simulink model "ModeAdjust"  (R2018b)
settings: Solver=FixedStepDiscrete  StartTime=0.0  StopTime=inf  FixedStep=0.01  RelTol=1e-3
undefined symbols (not defined in the file or in its folder): IfKeSMSbSeatMovBkRclnEnable_Val, IfKeSMSbSeatMovFrwdBkwdEnable_Val, IfKeSMSbSeatMovFtrstEnable_Val, IfKeSMSbSeatMovHdrstFrwdBkwdEnable_Val, IfKeSMSbSeatMovHdUpwdDnwdEnable_Val, IfKeSMSbSeatMovLgrstEnable_Val, IfKeSMSbSeatMovLtwdRtwdEnable_Val, IfVeSMSeStNumConfig, KeSMSbArmscreenMovEnable_Val, KeSMSbSeatMovLgrstExpdEnable_Val, KeSMSuFirstRwStBackPosDelta_Val, KeSMSuFirstRwStBackPosTolr_Val, KeSMSuFirstRwStCushFrntPosDelta_Val, KeSMSuFirstRwStCushFrntPosTolr_Val, KeSMSuFirstRwStCushRePosDelta_Val, KeSMSuFirstRwStCushRePosTolr_Val, KeSMSuFirstRwStFootrestPosDelta_Val, KeSMSuFirstRwStFootrestPosTolr_Val, KeSMSuFirstRwStFwdBkwdPosDelta_Val, KeSMSuFirstRwStFwdBkwdPosTolr_Val, KeSMSuMdMotFinshdTm_Val, KeSMSuMdRetryTm1_Val, KeSMSuModeReqDurgTm_Val, KeSMSuSecRwStArmTochPosDelta_Val, KeSMSuSecRwStArmTochPosTolr_Val, KeSMSuSecRwStBackPosDelta_Val, KeSMSuSecRwStBackPosTolr_Val, KeSMSuSecRwStFtrstUpwdDnwdPosDelta_Val, KeSMSuSecRwStFtrstUpwdDnwdPosTolr_Val, KeSMSuSecRwStFwdBkwdPosDelta_Val, KeSMSuSecRwStFwdBkwdPosTolr_Val, KeSMSuSecRwStHeadrestFwdBkwdPosDelta_Val, KeSMSuSecRwStHeadrestFwdBkwdPosTolr_Val, KeSMSuSecRwStHeadrestUpwdDwnwdPosDelta_Val, KeSMSuSecRwStHeadrestUpwdDwnwdPosTolr_Val, KeSMSuSecRwStLegrestInOutPosDelta_Val, KeSMSuSecRwStLegrestInOutPosTolr_Val, KeSMSuSecRwStLegrestUpwdDwnwdPosDelta_Val, KeSMSuSecRwStLegrestUpwdDwnwdPosTolr_Val, KeSMSuSecRwStLwdRwdPosDelta_Val, KeSMSuSecRwStLwdRwdPosTolr_Val, KeSMSuSecRwStVIPFtrstRefAngle_Val, KeSMSuThirdRwStFwdBkwdPosDelta_Val, KeSMSuThirdRwStFwdBkwdPosTolr_Val, KeSMSuThrdRwCushFoldPosDelta_Val, KeSMSuThrdRwCushFoldPosTolr_Val, KeSMSuThrdRwStBackPosDelta_Val, KeSMSuThrdRwStBackPosTolr_Val, KeSMSw4SLegrstCloseMdSecRwLtStFtrstUpwdDnwdPos_Val, KeSMSw4SLegrstCloseMdSecRwLtStFtrstUpwdDnwdPosMax_Val, KeSMSw4SLegrstCloseMdSecRwLtStFtrstUpwdDnwdPosMin_Val, KeSMSw4SLegrstCloseMdSecRwLtStLgrstOtwdInwdPos_Val, KeSMSw4SLegrstCloseMdSecRwLtStLgrstOtwdInwdPosMax_Val, KeSMSw4SLegrstCloseMdSecRwLtStLgrstOtwdInwdPosMin_Val, KeSMSw4SLegrstCloseMdSecRwLtStLgrstUpwdDnwdPos_Val, KeSMSw4SLegrstCloseMdSecRwLtStLgrstUpwdDnwdPosMax_Val, KeSMSw4SLegrstCloseMdSecRwLtStLgrstUpwdDnwdPosMin_Val, KeSMSw4SLegrstCloseMdSecRwRtStFtrstUpwdDnwdPos_Val, KeSMSw4SLegrstCloseMdSecRwRtStFtrstUpwdDnwdPosMax_Val, KeSMSw4SLegrstCloseMdSecRwRtStFtrstUpwdDnwdPosMin_Val ... (+1138)
libraries: Lib x401
(part 1 of 35)
settings Model: PauseTimes=0.02  TunableVars=ArmScrnDisable  TunableVarsStorageClass=ExportedGlobal  TunableVarsTypeQualifier=const  Creator=huanglu  LastModifiedBy=sn2xws
settings Model: ModifiedComment=|
  | sn2xws -- Mon Feb 20 10:45:59 2023 -- Version MY25 V1.4.0
  | Change Request 324651
settings Model: ModifiedHistory=|
  | sn2xws -- Mon Feb 20 10:45:59 2023 -- Version MY25 V1.4.0
  | Change Request 324651
  | 增加tlor标定，用于判断模式调用成功与否
  | 
  | 
  | 
  | sn2xws -- Thu Jan 05 09:24:50 2023 -- Version 2.7.0
  | 修改腿托系统打开闭合的流程
  | 
  | sn2xws -- Wed Apr 27 10:37:37 2022 -- Version 1.7.1
  | 身高查表改为标定值，增加全躺自适应
  | 
  | sn2xws -- Fri Feb 11 08:02:27 2022 -- Version 1.6.1
  | 增加vip4s 头枕腿托自适应功能
  | 
  | sn2xws -- Wed Jan 05 13:00:10 2022-- Version 1.5.2
  | bug 197485 二排单侧无人乘坐时，三排长滑轨速度命令不正确，
  | 三排左右速度信号连接反了已修复
  | 
  | sn2xws -- Tue Nov 30 10:28:27 2021 -- Version 1.5.1
  | 右侧扶手屏配置信号恢复连接
  | 删除无用输入接口
  | 增加亲密模式右
  | 增加腿托一键打开，一键关闭模式
  | CR134222：更新需求417/640/633/638 增加模式滑轨速度
  | CR179276 修改亲密模式，照顾模式，4s复位模式流程
  | 
  | sn2xws -- Mon Oct 18 17:11:57 2021 -- Version 1.3.5.9
  | closedownpos1,closedownpos2写反改正
  | sn2xws -- Wed Oct 13 15:34:21 2021 -- Version 1.3.5.8
  | 修改是否是四座版判断，增加上4p枚举
  | sn2xws -- Wed Oct 13 15:33:22 2021 -- Version 1.3.5.8
  | 将eze模式脚蹬改到第二阶段
  | 
  | delete vip CshnFld for coverage
  | 
  | for coverage outnumR3_R delete 2
  | code for float
  | sn2xws -- Tue Sep 07 13:48:55 2021 -- Version 1.3.5.7
  | 亲密模式和照顾模式不看童锁
  | 
  | sn2xws -- Fri Aug 27 15:43:38 2021 -- Version 1.3.5.6
  | cr 155453
  | 四座版模式流程修改，增加头枕前后
  | 
  | sn2xws -- Wed Aug 18 15:34:52 2021 -- Version 1.3.5.5
  | 进入模式二排做前后在位置判断连线错误修改
  | 
  | sn2xws -- Wed Aug 18 12:47:39 2021 -- Version 1.3.5.5
  | eze目标位置判断1排脚蹬配置信号连错修改
  | 
  | 
  | sn2xws -- Mon Aug 16 13:49:15 2021 -- Version 1.3.5.4
  | 扶手屏配置信号被占用，短措改为始终配置
  | 
  | sn2xws -- Wed Aug 11 15:50:26 2021 -- Version 1.3.5.3
  | 1.Change Request 147541L：更改7S版本VIP L的模式流程，删除三排右侧动作
  | 2.调用成功的前提条件修改，原先必须到目标位置，改成到目标区域
  | 3.在目标区域逻辑优化，增加valid判断,eze增加hold、占座判断
  | 
  | 
  | sn2xws -- Wed Aug 11 15:48:36 2021 -- Version 1.3.5.2
  | 修改4s腿托一键闭合流程中标定，closedownpos2改为closedownpos1
  | 
  | sn2xws -- Fri Aug 06 13:02:13 2021 -- Version 1.3.5.1
  | 210806:
  | 1.修正各模式童锁条件，等于lock改为不等于unlock
  | 2.family和intm模式增加童锁退出模式条件
settings DataIOCC: SaveFormat=StructureWithTime  ReturnWorkspaceOutputs=on
settings OptimizationCC: DefaultParameterBehavior=Inlined  EnhancedBackFolding=on  PassReuseOutputArgsAs=Individual arguments  ZeroExternalMemoryAtStartup=off  ZeroInternalMemoryAtStartup=off  OptimizeBlockOrder=speed  DifferentSizesBufferReuse=on  OptimizationCustomize=off
settings DebuggingCC: ParameterTunabilityLossMsg=error
settings HardwareCC: ProdBitPerPointer=32  ProdBitPerSizeT=32  ProdBitPerPtrDiffT=32  ProdLargestAtomicFloat=Double  ProdWordSize=32  ProdHWDeviceType=Renesas->RH850
settings ModelReferenceCC: ModelReferenceNumInstancesAllowed=Single
settings SFSimCC: SimCustomHeaderCode="#include\"Rte_Type.h\""  MATLABDynamicMemAlloc=off
settings RTWCC: SystemTargetFile=autosar.tlc  GenCodeOnly=on  TemplateMakefile=ert_default_tmf  Description=AUTOSAR  GenerateReport=on  IncludeHyperlinkInReport=on  LaunchReport=on  CodeExecutionProfiling=on  GenerateTraceInfo=on  GenerateTraceReport=on  GenerateTraceReportSl=on  GenerateTraceReportSf=on  GenerateTraceReportEml=on  GenerateCodeMetricsReport=on
settings CodeAppCC: ForceParamTrailComments=on  IgnoreCustomStorageClasses=off  MaxIdLength=63  OperatorAnnotations=on  SimulinkDataObjDesc=on  SFDataObjDesc=on  InsertBlockDesc=on
settings STFCustomTargetCC: TargetLangStandard=C99 (ISO)  MultiwordLength=256  ParMdlRefBuildCompliant=on  CompOptLevelCompliant=on  IncludeMdlTerminateFcn=off  CombineOutputUpdateFcns=on  SuppressErrorStatus=on  ERTCustomFileBanners=on  SupportAbsoluteTime=off  SupportNonFinite=off  SupportComplex=off  SupportContinuousTime=off  SupportNonInlinedSFcns=off  RemoveResetFunc=on  MATLABClassNameForMDSCustomization=Simulink.SoftwareTarget.ERTCustomization  AutosarCompliant=on  UseToolchainInfoCompliant=on  LookupTableObjectStructAxisOrder=2,1,3,4,...  LUTObjectStructOrderEvenSpacing=Size,Table,Breakpoints  SystemTargetFile=autosar.tlc
settings ERTTargetCC: TargetLangStandard=C99 (ISO)  ConcurrentExecutionCompliant=off  IncludeMdlTerminateFcn=off  SuppressErrorStatus=on  SupportAbsoluteTime=off  SupportNonFinite=off  SupportComplex=off  ModelStepFunctionPrototypeControlCompliant=off  CPPClassGenCompliant=off  AutosarCompliant=on  LookupTableObjectStructAxisOrder=2,1,3,4,...  LUTObjectStructOrderEvenSpacing=Size,Table,Breakpoints  ERTCustomFileTemplate=example_file_process.tlc  ERTFilePackagingFormat=Compact
settings ConfigComp: DVTestSuiteOptimization=CombinedObjectives (Nonlinear Extended)  DVDetectActiveLogic=on  DVDetectOutOfBounds=on

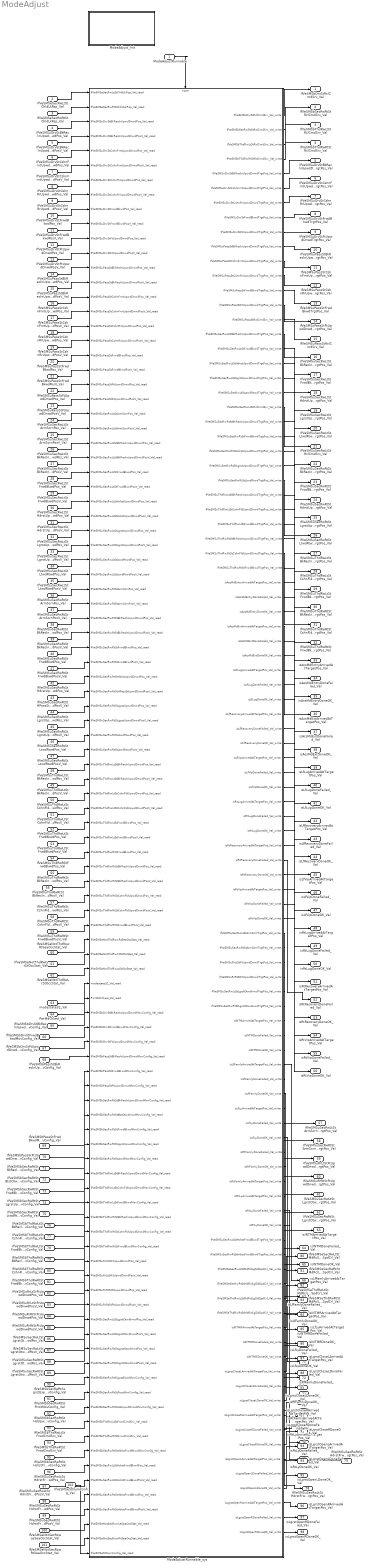
== system ModeAdjust ==
  ModeAdjustRunnable : Inport  SampleTime=0.01  OutputFunctionCall=on
  IfVeSMSeSecRwLtStChldLkRsp_Val : Inport  Port=2  OutDataTypeStr=Enum: SeatChldLkSt  PortDimensions=1
  IfVeSMSeSecRwRtStChldLkRsp_Val : Inport  Port=3  OutDataTypeStr=Enum: SeatChldLkSt  PortDimensions=1
  IfVeSMSuDrvStBkReclnUpwdDnwdPos_Val : Inport  Port=4  OutDataTypeStr=uint16  PortDimensions=1
  IfVeSMSuDrvStBkReclnUpwdDnwdPosV_Val : Inport  Port=5  OutDataTypeStr=boolean  PortDimensions=1
  IfVeSMSuDrvStCshnFrntUpwdDnwdPos_Val : Inport  Port=6  OutDataTypeStr=uint16  PortDimensions=1
  IfVeSMSuDrvStCshnFrntUpwdDnwdPosV_Val : Inport  Port=7  OutDataTypeStr=boolean  PortDimensions=1
  IfVeSMSuDrvStCshnRrUpwdDnwdPos_Val : Inport  Port=8  OutDataTypeStr=uint16  PortDimensions=1
  IfVeSMSuDrvStCshnRrUpwdDnwdPosV_Val : Inport  Port=9  OutDataTypeStr=boolean  PortDimensions=1
  IfVeSMSuDrvStFrwdBkwdPos_Val : Inport  Port=10  OutDataTypeStr=uint16  PortDimensions=1
  IfVeSMSuDrvStFrwdBkwdPosV_Val : Inport  Port=11  OutDataTypeStr=boolean  PortDimensions=1
  IfVeSMSuDrvStFtUpwdDnwdPos_Val : Inport  Port=12  OutDataTypeStr=uint16  PortDimensions=1
  IfVeSMSuDrvStFtUpwdDnwdPosV_Val : Inport  Port=13  OutDataTypeStr=boolean  PortDimensions=1
  IfVeSMSuPassStBkReclnUpwdDnwdPos_Val : Inport  Port=14  OutDataTypeStr=uint16  PortDimensions=1
  IfVeSMSuPassStBkReclnUpwdDnwdPosV_Val : Inport  Port=15  OutDataTypeStr=boolean  PortDimensions=1
  IfVeSMSuPassStCshnFrntUpwdDnwdPos_Val : Inport  Port=16  OutDataTypeStr=uint16  PortDimensions=1
  IfVeSMSuPassStCshnFrntUpwdDnwdPosV_Val : Inport  Port=17  OutDataTypeStr=boolean  PortDimensions=1
  IfVeSMSuPassStCshnRrUpwdDnwdPos_Val : Inport  Port=18  OutDataTypeStr=uint16  PortDimensions=1
  IfVeSMSuPassStCshnRrUpwdDnwdPosV_Val : Inport  Port=19  OutDataTypeStr=boolean  PortDimensions=1
  IfVeSMSuPassStFrwdBkwdPos_Val : Inport  Port=20  OutDataTypeStr=uint16  PortDimensions=1
  IfVeSMSuPassStFrwdBkwdPosV_Val : Inport  Port=21  OutDataTypeStr=boolean  PortDimensions=1
  IfVeSMSuPassStFtUpwdDnwdPos_Val : Inport  Port=22  OutDataTypeStr=uint16  PortDimensions=1
  IfVeSMSuPassStFtUpwdDnwdPosV_Val : Inport  Port=23  OutDataTypeStr=boolean  PortDimensions=1
  IfVeSMSuSecRwLtStArmScrnPos_Val : Inport  Port=24  OutDataTypeStr=uint16  PortDimensions=1
  IfVeSMSuSecRwLtStArmScrnPosV_Val : Inport  Port=25  OutDataTypeStr=boolean  PortDimensions=1
  IfVeSMSuSecRwLtStBkReclnUpwdDnwdPos_Val : Inport  Port=26  OutDataTypeStr=uint16  PortDimensions=1
  IfVeSMSuSecRwLtStBkReclnUpwdDnwdPosV_Val : Inport  Port=27  OutDataTypeStr=boolean  PortDimensions=1
  IfVeSMSuSecRwLtStFrwdBkwdPos_Val : Inport  Port=28  OutDataTypeStr=uint16  PortDimensions=1
  IfVeSMSuSecRwLtStFrwdBkwdPosV_Val : Inport  Port=29  OutDataTypeStr=boolean  PortDimensions=1
  IfVeSMSuSecRwLtStHdrstUpwdDnwdPos_Val : Inport  Port=30  OutDataTypeStr=uint16  PortDimensions=1
  IfVeSMSuSecRwLtStHdrstUpwdDnwdPosV_Val : Inport  Port=31  OutDataTypeStr=boolean  PortDimensions=1
  IfVeSMSuSecRwLtStLgrstUpwdDnwdPos_Val : Inport  Port=32  OutDataTypeStr=uint16  PortDimensions=1
  IfVeSMSuSecRwLtStLgrstUpwdDnwdPosV_Val : Inport  Port=33  OutDataTypeStr=boolean  PortDimensions=1
  IfVeSMSuSecRwLtStLtwdRtwdPos_Val : Inport  Port=34  OutDataTypeStr=uint16  PortDimensions=1
  IfVeSMSuSecRwLtStLtwdRtwdPosV_Val : Inport  Port=35  OutDataTypeStr=boolean  PortDimensions=1
  IfVeSMSuSecRwRtStArmScrnPos_Val : Inport  Port=36  OutDataTypeStr=uint16  PortDimensions=1
  IfVeSMSuSecRwRtStArmScrnPosV_Val : Inport  Port=37  OutDataTypeStr=boolean  PortDimensions=1
  IfVeSMSuSecRwRtStBkReclnUpwdDnwdPos_Val : Inport  Port=38  OutDataTypeStr=uint16  PortDimensions=1
  IfVeSMSuSecRwRtStBkReclnUpwdDnwdPosV_Val : Inport  Port=39  OutDataTypeStr=boolean  PortDimensions=1
  IfVeSMSuSecRwRtStFrwdBkwdPos_Val : Inport  Port=40  OutDataTypeStr=uint16  PortDimensions=1
  IfVeSMSuSecRwRtStFrwdBkwdPosV_Val : Inport  Port=41  OutDataTypeStr=boolean  PortDimensions=1
  IfVeSMSuSecRwRtStHdrstUpwdDnwdPos_Val : Inport  Port=42  OutDataTypeStr=uint16  PortDimensions=1
  IfVeSMSuSecRwRtStHPassStUpwdDnwdPosV_Val : Inport  Port=43  OutDataTypeStr=boolean  PortDimensions=1
  IfVeSMSuSecRwRtStLgrstUpwdDnwdPos_Val : Inport  Port=44  OutDataTypeStr=uint16  PortDimensions=1
  IfVeSMSuSecRwRtStLgrstUpwdDnwdPosV_Val : Inport  Port=45  OutDataTypeStr=boolean  PortDimensions=1
  IfVeSMSuSecRwRtStLtwdRtwdPos_Val : Inport  Port=46  OutDataTypeStr=uint16  PortDimensions=1
  IfVeSMSuSecRwRtStLtwdRtwdPosV_Val : Inport  Port=47  OutDataTypeStr=boolean  PortDimensions=1
  IfVeSMSuThdRwLtStBkReclnUpwdDnwdPos_Val : Inport  Port=48  OutDataTypeStr=uint16  PortDimensions=1
  IfVeSMSuThdRwLtStBkReclnUpwdDnwdPosV_Val : Inport  Port=49  OutDataTypeStr=boolean  PortDimensions=1
  IfVeSMSuThdRwLtStCshnFldUpwdDnwdPos_Val : Inport  Port=50  OutDataTypeStr=uint16  PortDimensions=1
  IfVeSMSuThdRwLtStCshnFldUpwdDnwdPosV_Val : Inport  Port=51  OutDataTypeStr=boolean  PortDimensions=1
  IfVeSMSuThdRwLtStFrwdBkwdPos_Val : Inport  Port=52  OutDataTypeStr=uint16  PortDimensions=1
  IfVeSMSuThdRwLtStFrwdBkwdPosV_Val : Inport  Port=53  OutDataTypeStr=boolean  PortDimensions=1
  IfVeSMSuThdRwRStFrwdBkwdPos_Val : Inport  Port=54  OutDataTypeStr=uint16  PortDimensions=1
  IfVeSMSuThdRwRtStBkReclnUpwdDnwdPos_Val : Inport  Port=55  OutDataTypeStr=uint16  PortDimensions=1
  IfVeSMSuThdRwRtStBkReclnUpwdDnwdPosV_Val : Inport  Port=56  OutDataTypeStr=boolean  PortDimensions=1
  IfVeSMSuThdRwRtStCshnFldUpwdDnwdPos_Val : Inport  Port=57  OutDataTypeStr=uint16  PortDimensions=1
  IfVeSMSuThdRwRtStCshnFldUpwdDnwdPosV_Val : Inport  Port=58  OutDataTypeStr=boolean  PortDimensions=1
  IfVeSMSuThdRwRtStFrwdBkwdPosV_Val : Inport  Port=59  OutDataTypeStr=boolean  PortDimensions=1
  IfVeSMSeNotThdRowRtSeaOccStat_Val : Inport  Port=60  OutDataTypeStr=Enum: SeatOccupiedSts1  PortDimensions=1
  IfVeSMSeNotThdRwCtStOccStat_Val : Inport  Port=61  OutDataTypeStr=Enum: SeatOccupiedSts1  PortDimensions=1
  IfVeSMSeNotThdRwLtStOccStat_Val : Inport  Port=62  OutDataTypeStr=Enum: SeatOccupiedSts1  PortDimensions=1
  modestate32_Val : Inport  Port=63  OutDataTypeStr=uint32  PortDimensions=1
  PwrMdChked_Val : Inport  Port=64  OutDataTypeStr=Enum: PowerMode1  PortDimensions=1
  IfVeSMSbDrvStBkReclnUpwdDnwdMovConfig_Val : Inport  Port=65  OutDataTypeStr=boolean  PortDimensions=1
  IfVeSMSbDrvStFrwdBkwdMovConfig_Val : Inport  Port=66  OutDataTypeStr=boolean  PortDimensions=1
  IfVeSMSbDrvStFtUpwdDnwdMovConfig_Val : Inport  Port=67  OutDataTypeStr=boolean  PortDimensions=1
  IfVeSMSbPassStBkReclnUpwdDnwdMovConfig_Val : Inport  Port=68  OutDataTypeStr=boolean  PortDimensions=1
  IfVeSMSbPassStFrwdBkwdMovConfig_Val : Inport  Port=69  OutDataTypeStr=boolean  PortDimensions=1
  IfVeSMSbPassStFtUpwdDnwdMovConfig_Val : Inport  Port=70  OutDataTypeStr=boolean  PortDimensions=1
  IfVeSMSbSecRwRtStBkReclnUpwdDnwdMovConfig_Val : Inport  Port=71  OutDataTypeStr=boolean  PortDimensions=1
  IfVeSMSbSecRwRtStBlstOtwdInwdMovConfig_Val : Inport  Port=72  OutDataTypeStr=boolean  PortDimensions=1
  IfVeSMSbSecRwRtStFrwdBkwdMovConfig_Val : Inport  Port=73  OutDataTypeStr=boolean  PortDimensions=1
  IfVeSMSbSecRwRtStLgrstUpwdMovConfig_Val : Inport  Port=74  OutDataTypeStr=boolean  PortDimensions=1
  IfVeSMSbSecRwRtStLtwdRtwdMovConfig_Val : Inport  Port=75  OutDataTypeStr=boolean  PortDimensions=1
  IfVeSMSbThdRwLtStBkReclnUpwdDnwdMovConfig_Val : Inport  Port=76  OutDataTypeStr=boolean  PortDimensions=1
  IfVeSMSbThdRwLtStCshnFldUpwdDnwdMovConfig_Val : Inport  Port=77  OutDataTypeStr=boolean  PortDimensions=1
  IfVeSMSbThdRwLtStFrwdBkwdMovConfig_Val : Inport  Port=78  OutDataTypeStr=boolean  PortDimensions=1
  IfVeSMSbThdRwRtStBkReclnUpwdDnwdMovConfig_Val : Inport  Port=79  OutDataTypeStr=boolean  PortDimensions=1
  IfVeSMSbThdRwRtStCshnFldUpwdDnwdMovConfig_Val : Inport  Port=80  OutDataTypeStr=boolean  PortDimensions=1
  IfVeSMSbThdRwRtStFrwdBkwdMovConfig_Val : Inport  Port=81  OutDataTypeStr=boolean  PortDimensions=1
  IfVeSMSuRrLtStFtUpwdDnwdPos_Val : Inport  Port=82  OutDataTypeStr=uint16  PortDimensions=1
  IfVeSMSuRrLtStFtUpwdDnwdPosV_Val : Inport  Port=83  OutDataTypeStr=boolean  PortDimensions=1
  IfVeSMSuRrRtStFtUpwdDnwdPos_Val : Inport  Port=84  OutDataTypeStr=uint16  PortDimensions=1
  IfVeSMSuRrRtStFtUpwdDnwdPosV_Val : Inport  Port=85  OutDataTypeStr=boolean  PortDimensions=1
  IfVeSMSuSecRwLtStLgrstOtwdInwdPos_Val : Inport  Port=86  OutDataTypeStr=uint16  PortDimensions=1
  IfVeSMSuSecRwLtStLgrstOtwdInwdPosV_Val : Inport  Port=87  OutDataTypeStr=boolean  PortDimensions=1
  IfVeSMSuSecRwRtStLgrstOtwdInwdPos_Val : Inport  Port=88  OutDataTypeStr=uint16  PortDimensions=1
  IfVeSMSuSecRwRtStLgrstOtwdInwdPosV_Val : Inport  Port=89  OutDataTypeStr=boolean  PortDimensions=1
  IfVeSMSbSecRwRtSLgrstExpdMovConfig_Val : Inport  Port=90  OutDataTypeStr=boolean  PortDimensions=1
  IfVeSMSbSecRwRtStFtrstMovConfig_Val : Inport  Port=91  OutDataTypeStr=boolean  PortDimensions=1
  IfVeSMSbSecRwRtStHdUpwdDnwdMovConfig_Val : Inport  Port=92  OutDataTypeStr=boolean  PortDimensions=1
  IfVeSMSbThdRwLtStFrwdCmdSrv_Val : Inport  Port=93  OutDataTypeStr=boolean  PortDimensions=1
  IfVeSMSbThdRwRtStFrwdCmdSrv_Val : Inport  Port=94  OutDataTypeStr=boolean  PortDimensions=1
  IfVeSMSbSecRwRtStHdrstFrwdBkwdMovConfig_Val : Inport  Port=95  OutDataTypeStr=boolean  PortDimensions=1
  IfVeSMSuSecRwLtStHdrstFrwdBkwdPos_Val : Inport  Port=96  OutDataTypeStr=uint16  PortDimensions=1
  IfVeSMSuSecRwLtStHdrstFrwdBkwdPosV_Val : Inport  Port=97  OutDataTypeStr=boolean  PortDimensions=1
  IfVeSMSuSecRwRtStHdrstFrwdBkwdPos_Val : Inport  Port=98  OutDataTypeStr=uint16  PortDimensions=1
  IfVeSMSuSecRwRtStHdrstFrwdBkwdPosV_Val : Inport  Port=99  OutDataTypeStr=boolean  PortDimensions=1
  IfVeSMSeNotSecRowLeSeaOccStat_Val : Inport  Port=100  OutDataTypeStr=Enum: SeatOccupiedSts1  PortDimensions=1
  IfVeSMSeNotSecRowRtSeaOccStat_Val : Inport  Port=101  OutDataTypeStr=Enum: SeatOccupiedSts1  PortDimensions=1
  IfVeSMSeStNumConfig_Val : Inport  Port=102  OutDataTypeStr=Enum: IfVeSMSeStNumConfig  PortDimensions=1
  ModeAdjustRunnable_sys : Subsystem
  ModeAdjust_Init : Subsystem
  IfVeSMSbDrvStRclCmdSrv_Val : Outport  OutDataTypeStr=boolean  PortDimensions=1
  IfVeSMSbSecRwRtStRclCmdSrv_Val : Outport  Port=2  OutDataTypeStr=boolean  PortDimensions=1
  IfVeSMSbThdRwLtStRclCmdSrv_Val : Outport  Port=3  OutDataTypeStr=boolean  PortDimensions=1
  IfVeSMSbThdRwRtStRclCmdSrv_Val : Outport  Port=4  OutDataTypeStr=boolean  PortDimensions=1
  IfVeSMSuDrvStBkReclnUpwdDnwdTrgtPos_Val : Outport  Port=5  OutDataTypeStr=uint16  PortDimensions=1
  IfVeSMSuDrvStCshnFrntUpwdDnwdTrgtPos_Val : Outport  Port=6  OutDataTypeStr=uint16  PortDimensions=1
  IfVeSMSuDrvStCshnRrUpwdDnwdTrgtPos_Val : Outport  Port=7  OutDataTypeStr=uint16  PortDimensions=1
  IfVeSMSuDrvStFrwdBkwdTrgtPos_Val : Outport  Port=8  OutDataTypeStr=uint16  PortDimensions=1
  IfVeSMSuDrvStFtUpwdDnwdTrgtPos_Val : Outport  Port=9  OutDataTypeStr=uint16  PortDimensions=1
  IfVeSMSuPassStBkReclnUpwdDnwdTrgtPos_Val : Outport  Port=10  OutDataTypeStr=uint16  PortDimensions=1
  IfVeSMSuPassStCshnFrntUpwdDnwdTrgtPos_Val : Outport  Port=11  OutDataTypeStr=uint16  PortDimensions=1
  IfVeSMSuPassStCshnRrUpwdDnwdTrgtPos_Val : Outport  Port=12  OutDataTypeStr=uint16  PortDimensions=1
  IfVeSMSuPassStFrwdBkwdTrgtPos_Val : Outport  Port=13  OutDataTypeStr=uint16  PortDimensions=1
  IfVeSMSuPassStFtUpwdDnwdTrgtPos_Val : Outport  Port=14  OutDataTypeStr=uint16  PortDimensions=1
  IfVeSMSuPassStRclCmdSrv_Val : Outport  Port=15  OutDataTypeStr=boolean  PortDimensions=1
  IfVeSMSuSecRwLtStBkReclnUpwdDnwdTrgtPos_Val : Outport  Port=16  OutDataTypeStr=uint16  PortDimensions=1
  IfVeSMSuSecRwLtStFrwdBkwdTrgtPos_Val : Outport  Port=17  OutDataTypeStr=uint16  PortDimensions=1
  IfVeSMSuSecRwLtStHdrstUpwdDnwdTrgtPos_Val : Outport  Port=18  OutDataTypeStr=uint16  PortDimensions=1
  IfVeSMSuSecRwLtStLgrstUpwdDnwdTrgtPos_Val : Outport  Port=19  OutDataTypeStr=uint16  PortDimensions=1
  IfVeSMSuSecRwLtStLtwdRtwdTrgtPos_Val : Outport  Port=20  OutDataTypeStr=uint16  PortDimensions=1
  IfVeSMSuSecRwLtStRclCmdSrv_Val : Outport  Port=21  OutDataTypeStr=boolean  PortDimensions=1
  IfVeSMSuSecRwRtStBkReclnUpwdDnwdTrgtPos_Val : Outport  Port=22  OutDataTypeStr=uint16  PortDimensions=1
  IfVeSMSuSecRwRtStFrwdBkwdTrgtPos_Val : Outport  Port=23  OutDataTypeStr=uint16  PortDimensions=1
  IfVeSMSuSecRwRtStHdrstUpwdDnwdTrgtPos_Val : Outport  Port=24  OutDataTypeStr=uint16  PortDimensions=1
  IfVeSMSuSecRwRtStLgrstUpwdDnwdTrgtPos_Val : Outport  Port=25  OutDataTypeStr=uint16  PortDimensions=1
  IfVeSMSuSecRwRtStLtwdRtwdTrgtPos_Val : Outport  Port=26  OutDataTypeStr=uint16  PortDimensions=1
  IfVeSMSuThdRwLtStBkReclnUpwdDnwdTrgtPos_Val : Outport  Port=27  OutDataTypeStr=uint16  PortDimensions=1
  IfVeSMSuThdRwLtStCshnFldUpwdDnwdTrgtPos_Val : Outport  Port=28  OutDataTypeStr=uint16  PortDimensions=1
  IfVeSMSuThdRwLtStFrwdBkwdTrgtPos_Val : Outport  Port=29  OutDataTypeStr=uint16  PortDimensions=1
  IfVeSMSuThdRwRtStBkReclnUpwdDnwdTrgtPos_Val : Outport  Port=30  OutDataTypeStr=uint16  PortDimensions=1
  IfVeSMSuThdRwRtStCshnFldUpwdDnwdTrgtPos_Val : Outport  Port=31  OutDataTypeStr=uint16  PortDimensions=1
  IfVeSMSuThdRwRtStFrwdBkwdTrgtPos_Val : Outport  Port=32  OutDataTypeStr=uint16  PortDimensions=1
  isAcsMdEntryArrivedAtTargetPos_Val : Outport  Port=33  OutDataTypeStr=boolean  PortDimensions=1
  isAcsMdEntryDoneFailed_Val : Outport  Port=34  OutDataTypeStr=boolean  PortDimensions=1
  isAcsMdEntryDoneOK_Val : Outport  Port=35  OutDataTypeStr=boolean  PortDimensions=1
  isAcsMdExtArrivedAtTargetPos_Val : Outport  Port=36  OutDataTypeStr=boolean  PortDimensions=1
  isAcsMdExtDoneFailed_Val : Outport  Port=37  OutDataTypeStr=boolean  PortDimensions=1
  isAcsMdExtDoneOK_Val : Outport  Port=38  OutDataTypeStr=boolean  PortDimensions=1
  isLfLugArrivedAtTargetPos_Val : Outport  Port=39  OutDataTypeStr=boolean  PortDimensions=1
  isLfLugDoneFailed_Val : Outport  Port=40  OutDataTypeStr=boolean  PortDimensions=1
  isLfLugDoneOK_Val : Outport  Port=41  OutDataTypeStr=boolean  PortDimensions=1
  isLfRecoveryArrivedAtTargetPos_Val : Outport  Port=42  OutDataTypeStr=boolean  PortDimensions=1
  isLfRecoveryDoneFailed_Val : Outport  Port=43  OutDataTypeStr=boolean  PortDimensions=1
  isLfRecoveryDoneOK_Val : Outport  Port=44  OutDataTypeStr=boolean  PortDimensions=1
  isLfVipArrivedAtTargetPos_Val : Outport  Port=45  OutDataTypeStr=boolean  PortDimensions=1
  isLfVipDoneFailed_Val : Outport  Port=46  OutDataTypeStr=boolean  PortDimensions=1
  isLfVipDoneOK_Val : Outport  Port=47  OutDataTypeStr=boolean  PortDimensions=1
  isRtLugArrivedAtTargetPos_Val : Outport  Port=48  OutDataTypeStr=boolean  PortDimensions=1
  isRtLugDoneFailed_Val : Outport  Port=49  OutDataTypeStr=boolean  PortDimensions=1
  isRtLugDoneOK_Val : Outport  Port=50  OutDataTypeStr=boolean  PortDimensions=1
  isRtRecoveryArrivedAtTargetPos_Val : Outport  Port=51  OutDataTypeStr=boolean  PortDimensions=1
  isRtRecoveryDoneFailed_Val : Outport  Port=52  OutDataTypeStr=boolean  PortDimensions=1
  isRtRecoveryDoneOK_Val : Outport  Port=53  OutDataTypeStr=boolean  PortDimensions=1
  isRtVipArrivedAtTargetPos_Val : Outport  Port=54  OutDataTypeStr=boolean  PortDimensions=1
  isRtVipDoneFailed_Val : Outport  Port=55  OutDataTypeStr=boolean  PortDimensions=1
  isRtVipDoneOK_Val : Outport  Port=56  OutDataTypeStr=boolean  PortDimensions=1
  IfVeSMSuSecRwLtStArmScrnTrgtPos_Val : Outport  Port=57  OutDataTypeStr=uint16  PortDimensions=1
  IfVeSMSuSecRwRtStArmScrnTrgtPos_Val : Outport  Port=58  OutDataTypeStr=uint16  PortDimensions=1
  IfVeSMSuRrLtStFtUpwdDnwdTrgtPos_Val : Outport  Port=59  OutDataTypeStr=uint16  PortDimensions=1
  IfVeSMSuRrRtStFtUpwdDnwdTrgtPos_Val : Outport  Port=60  OutDataTypeStr=uint16  PortDimensions=1
  IfVeSMSuSecRwLtStLgrstOtwdInwdTrgtPos_Val : Outport  Port=61  OutDataTypeStr=uint16  PortDimensions=1
  IfVeSMSuSecRwRtStLgrstOtwdInwdTrgtPos_Val : Outport  Port=62  OutDataTypeStr=uint16  PortDimensions=1
  isINTMArrivedAtTargetPos_Val : Outport  Port=63  OutDataTypeStr=boolean  PortDimensions=1
  isINTMDoneFailed_Val : Outport  Port=64  OutDataTypeStr=boolean  PortDimensions=1
  isINTMDoneOK_Val : Outport  Port=65  OutDataTypeStr=boolean  PortDimensions=1
  isLfFamlyArrivedAtTargetPos_Val : Outport  Port=66  OutDataTypeStr=boolean  PortDimensions=1
  isLfFamlyDoneFailed_Val : Outport  Port=67  OutDataTypeStr=boolean  PortDimensions=1
  isLfFamlyDoneOK_Val : Outport  Port=68  OutDataTypeStr=boolean  PortDimensions=1
  isLfLyArrivedAtTargetPos_Val : Outport  Port=69  OutDataTypeStr=boolean  PortDimensions=1
  isLfLyDoneFailed_Val : Outport  Port=70  OutDataTypeStr=boolean  PortDimensions=1
  isLfLyDoneOK_Val : Outport  Port=71  OutDataTypeStr=boolean  PortDimensions=1
  isRfFamlyDoneFailed_Val : Outport  Port=72  OutDataTypeStr=boolean  PortDimensions=1
  isRfFamlyDoneOK_Val : Outport  Port=73  OutDataTypeStr=boolean  PortDimensions=1
  isRtFamlyArrivedAtTargetPos_Val : Outport  Port=74  OutDataTypeStr=boolean  PortDimensions=1
  isRtLyArrivedAtTargetPos_Val : Outport  Port=75  OutDataTypeStr=boolean  PortDimensions=1
  isRtLyDoneFailed_Val : Outport  Port=76  OutDataTypeStr=boolean  PortDimensions=1
  isRtLyDoneOK_Val : Outport  Port=77  OutDataTypeStr=boolean  PortDimensions=1
  IfVeSMSuSecRwLtStHdrstFrwdBkwdTrgtPos_Val : Outport  Port=78  OutDataTypeStr=uint16  PortDimensions=1
  IfVeSMSuSecRwRtStHdrstFrwdBkwdTrgtPos_Val : Outport  Port=79  OutDataTypeStr=uint16  PortDimensions=1
  IfVeSMSeSecRwLtStMdRclLgSldSpdCrl_Val : Outport  Port=80  OutDataTypeStr=uint8  PortDimensions=1
  IfVeSMSeSecRwRtStMdRclLgSldSpdCrl_Val : Outport  Port=81  OutDataTypeStr=uint8  PortDimensions=1
  IfVeSMSeThdRwLtStMdRclLgSldSpdCrl_Val : Outport  Port=82  OutDataTypeStr=uint8  PortDimensions=1
  IfVeSMSeThdRwRtStMdRclLgSldSpdCrl_Val : Outport  Port=83  OutDataTypeStr=uint8  PortDimensions=1
  isINTMRArrivedAtTargetPos_Val : Outport  Port=84  OutDataTypeStr=boolean  PortDimensions=1
  isINTMRDoneFailed_Val : Outport  Port=85  OutDataTypeStr=boolean  PortDimensions=1
  isINTMRDoneOK_Val : Outport  Port=86  OutDataTypeStr=boolean  PortDimensions=1
  isLgrstCloseLArrivedAtTargetPos_Val : Outport  Port=87  OutDataTypeStr=boolean  PortDimensions=1
  isLgrstCloseLDoneFailed_Val : Outport  Port=88  OutDataTypeStr=boolean  PortDimensions=1
  isLgrstCloseLDoneOK_Val : Outport  Port=89  OutDataTypeStr=boolean  PortDimensions=1
  isLgrstCloseRArrivedAtTargetPos_Val : Outport  Port=90  OutDataTypeStr=boolean  PortDimensions=1
  isLgrstCloseRDoneFailed_Val : Outport  Port=91  OutDataTypeStr=boolean  PortDimensions=1
  isLgrstCloseRDoneOK_Val : Outport  Port=92  OutDataTypeStr=boolean  PortDimensions=1
  isLgrstOpenLArrivedAtTargetPos_Val : Outport  Port=93  OutDataTypeStr=boolean  PortDimensions=1
  isLgrstOpenLDoneFailed_Val : Outport  Port=94  OutDataTypeStr=boolean  PortDimensions=1
  isLgrstOpenLDoneOK_Val : Outport  Port=95  OutDataTypeStr=boolean  PortDimensions=1
  isLgrstOpenRArrivedAtTargetPos_Val : Outport  Port=96  OutDataTypeStr=boolean  PortDimensions=1
  isLgrstOpenRDoneFailed_Val : Outport  Port=97  OutDataTypeStr=boolean  PortDimensions=1
  isLgrstOpenRDoneOK_Val : Outport  Port=98  OutDataTypeStr=boolean  PortDimensions=1
  wires:
  IfVeSMSeSecRwLtStChldLkRsp_Val/1 -> ModeAdjustRunnable_sys/1(IfVeSMSeSecRwLtStChldLkRsp_Val_read)
  IfVeSMSeSecRwRtStChldLkRsp_Val/1 -> ModeAdjustRunnable_sys/2(IfVeSMSeSecRwRtStChldLkRsp_Val_read)
  IfVeSMSuDrvStBkReclnUpwdDnwdPos_Val/1 -> ModeAdjustRunnable_sys/3(IfVeSMSuDrvStBkReclnUpwdDnwdPos_Val_read)
  IfVeSMSuDrvStBkReclnUpwdDnwdPosV_Val/1 -> ModeAdjustRunnable_sys/4(IfVeSMSuDrvStBkReclnUpwdDnwdPosV_Val_read)
  IfVeSMSuDrvStCshnFrntUpwdDnwdPos_Val/1 -> ModeAdjustRunnable_sys/5(IfVeSMSuDrvStCshnFrntUpwdDnwdPos_Val_read)
  IfVeSMSuDrvStCshnFrntUpwdDnwdPosV_Val/1 -> ModeAdjustRunnable_sys/6(IfVeSMSuDrvStCshnFrntUpwdDnwdPosV_Val_read)
  IfVeSMSuDrvStCshnRrUpwdDnwdPos_Val/1 -> ModeAdjustRunnable_sys/7(IfVeSMSuDrvStCshnRrUpwdDnwdPos_Val_read)
  IfVeSMSuDrvStCshnRrUpwdDnwdPosV_Val/1 -> ModeAdjustRunnable_sys/8(IfVeSMSuDrvStCshnRrUpwdDnwdPosV_Val_read)
  IfVeSMSuDrvStFrwdBkwdPos_Val/1 -> ModeAdjustRunnable_sys/9(IfVeSMSuDrvStFrwdBkwdPos_Val_read)
  IfVeSMSuDrvStFrwdBkwdPosV_Val/1 -> ModeAdjustRunnable_sys/10(IfVeSMSuDrvStFrwdBkwdPosV_Val_read)
  IfVeSMSuDrvStFtUpwdDnwdPos_Val/1 -> ModeAdjustRunnable_sys/11(IfVeSMSuDrvStFtUpwdDnwdPos_Val_read)
  IfVeSMSuDrvStFtUpwdDnwdPosV_Val/1 -> ModeAdjustRunnable_sys/12(IfVeSMSuDrvStFtUpwdDnwdPosV_Val_read)
  IfVeSMSuPassStBkReclnUpwdDnwdPos_Val/1 -> ModeAdjustRunnable_sys/13(IfVeSMSuPassStBkReclnUpwdDnwdPos_Val_read)
  IfVeSMSuPassStBkReclnUpwdDnwdPosV_Val/1 -> ModeAdjustRunnable_sys/14(IfVeSMSuPassStBkReclnUpwdDnwdPosV_Val_read)
  IfVeSMSuPassStCshnFrntUpwdDnwdPos_Val/1 -> ModeAdjustRunnable_sys/15(IfVeSMSuPassStCshnFrntUpwdDnwdPos_Val_read)
  IfVeSMSuPassStCshnFrntUpwdDnwdPosV_Val/1 -> ModeAdjustRunnable_sys/16(IfVeSMSuPassStCshnFrntUpwdDnwdPosV_Val_read)
  IfVeSMSuPassStCshnRrUpwdDnwdPos_Val/1 -> ModeAdjustRunnable_sys/17(IfVeSMSuPassStCshnRrUpwdDnwdPos_Val_read)
  IfVeSMSuPassStCshnRrUpwdDnwdPosV_Val/1 -> ModeAdjustRunnable_sys/18(IfVeSMSuPassStCshnRrUpwdDnwdPosV_Val_read)
  IfVeSMSuPassStFrwdBkwdPos_Val/1 -> ModeAdjustRunnable_sys/19(IfVeSMSuPassStFrwdBkwdPos_Val_read)
  IfVeSMSuPassStFrwdBkwdPosV_Val/1 -> ModeAdjustRunnable_sys/20(IfVeSMSuPassStFrwdBkwdPosV_Val_read)
  IfVeSMSuPassStFtUpwdDnwdPos_Val/1 -> ModeAdjustRunnable_sys/21(IfVeSMSuPassStFtUpwdDnwdPos_Val_read)
  IfVeSMSuPassStFtUpwdDnwdPosV_Val/1 -> ModeAdjustRunnable_sys/22(IfVeSMSuPassStFtUpwdDnwdPosV_Val_read)
  IfVeSMSuSecRwLtStArmScrnPos_Val/1 -> ModeAdjustRunnable_sys/23(IfVeSMSuSecRwLtStArmScrnPos_Val_read)
  IfVeSMSuSecRwLtStArmScrnPosV_Val/1 -> ModeAdjustRunnable_sys/24(IfVeSMSuSecRwLtStArmScrnPosV_Val_read)
  IfVeSMSuSecRwLtStBkReclnUpwdDnwdPos_Val/1 -> ModeAdjustRunnable_sys/25(IfVeSMSuSecRwLtStBkReclnUpwdDnwdPos_Val_read)
  IfVeSMSuSecRwLtStBkReclnUpwdDnwdPosV_Val/1 -> ModeAdjustRunnable_sys/26(IfVeSMSuSecRwLtStBkReclnUpwdDnwdPosV_Val_read)
  IfVeSMSuSecRwLtStFrwdBkwdPos_Val/1 -> ModeAdjustRunnable_sys/27(IfVeSMSuSecRwLtStFrwdBkwdPos_Val_read)
  IfVeSMSuSecRwLtStFrwdBkwdPosV_Val/1 -> ModeAdjustRunnable_sys/28(IfVeSMSuSecRwLtStFrwdBkwdPosV_Val_read)
  IfVeSMSuSecRwLtStHdrstUpwdDnwdPos_Val/1 -> ModeAdjustRunnable_sys/29(IfVeSMSuSecRwLtStHdrstUpwdDnwdPos_Val_read)
  IfVeSMSuSecRwLtStHdrstUpwdDnwdPosV_Val/1 -> ModeAdjustRunnable_sys/30(IfVeSMSuSecRwLtStHdrstUpwdDnwdPosV_Val_read)
  IfVeSMSuSecRwLtStLgrstUpwdDnwdPos_Val/1 -> ModeAdjustRunnable_sys/31(IfVeSMSuSecRwLtStLgrstUpwdDnwdPos_Val_read)
  IfVeSMSuSecRwLtStLgrstUpwdDnwdPosV_Val/1 -> ModeAdjustRunnable_sys/32(IfVeSMSuSecRwLtStLgrstUpwdDnwdPosV_Val_read)
  IfVeSMSuSecRwLtStLtwdRtwdPos_Val/1 -> ModeAdjustRunnable_sys/33(IfVeSMSuSecRwLtStLtwdRtwdPos_Val_read)
  IfVeSMSuSecRwLtStLtwdRtwdPosV_Val/1 -> ModeAdjustRunnable_sys/34(IfVeSMSuSecRwLtStLtwdRtwdPosV_Val_read)
  IfVeSMSuSecRwRtStArmScrnPos_Val/1 -> ModeAdjustRunnable_sys/35(IfVeSMSuSecRwRtStArmScrnPos_Val_read)
  IfVeSMSuSecRwRtStArmScrnPosV_Val/1 -> ModeAdjustRunnable_sys/36(IfVeSMSuSecRwRtStArmScrnPosV_Val_read)
  IfVeSMSuSecRwRtStBkReclnUpwdDnwdPos_Val/1 -> ModeAdjustRunnable_sys/37(IfVeSMSuSecRwRtStBkReclnUpwdDnwdPos_Val_read)
  IfVeSMSuSecRwRtStBkReclnUpwdDnwdPosV_Val/1 -> ModeAdjustRunnable_sys/38(IfVeSMSuSecRwRtStBkReclnUpwdDnwdPosV_Val_read)
  IfVeSMSuSecRwRtStFrwdBkwdPos_Val/1 -> ModeAdjustRunnable_sys/39(IfVeSMSuSecRwRtStFrwdBkwdPos_Val_read)
  IfVeSMSuSecRwRtStFrwdBkwdPosV_Val/1 -> ModeAdjustRunnable_sys/40(IfVeSMSuSecRwRtStFrwdBkwdPosV_Val_read)
  IfVeSMSuSecRwRtStHdrstUpwdDnwdPos_Val/1 -> ModeAdjustRunnable_sys/41(IfVeSMSuSecRwRtStHdrstUpwdDnwdPos_Val_read)
  IfVeSMSuSecRwRtStHPassStUpwdDnwdPosV_Val/1 -> ModeAdjustRunnable_sys/42(IfVeSMSuSecRwRtStHPassStUpwdDnwdPosV_Val_read)
  IfVeSMSuSecRwRtStLgrstUpwdDnwdPos_Val/1 -> ModeAdjustRunnable_sys/43(IfVeSMSuSecRwRtStLgrstUpwdDnwdPos_Val_read)
  IfVeSMSuSecRwRtStLgrstUpwdDnwdPosV_Val/1 -> ModeAdjustRunnable_sys/44(IfVeSMSuSecRwRtStLgrstUpwdDnwdPosV_Val_read)
  IfVeSMSuSecRwRtStLtwdRtwdPos_Val/1 -> ModeAdjustRunnable_sys/45(IfVeSMSuSecRwRtStLtwdRtwdPos_Val_read)
  IfVeSMSuSecRwRtStLtwdRtwdPosV_Val/1 -> ModeAdjustRunnable_sys/46(IfVeSMSuSecRwRtStLtwdRtwdPosV_Val_read)
  IfVeSMSuThdRwLtStBkReclnUpwdDnwdPos_Val/1 -> ModeAdjustRunnable_sys/47(IfVeSMSuThdRwLtStBkReclnUpwdDnwdPos_Val_read)
  IfVeSMSuThdRwLtStBkReclnUpwdDnwdPosV_Val/1 -> ModeAdjustRunnable_sys/48(IfVeSMSuThdRwLtStBkReclnUpwdDnwdPosV_Val_read)
  IfVeSMSuThdRwLtStCshnFldUpwdDnwdPos_Val/1 -> ModeAdjustRunnable_sys/49(IfVeSMSuThdRwLtStCshnFldUpwdDnwdPos_Val_read)
  IfVeSMSuThdRwLtStCshnFldUpwdDnwdPosV_Val/1 -> ModeAdjustRunnable_sys/50(IfVeSMSuThdRwLtStCshnFldUpwdDnwdPosV_Val_read)
  IfVeSMSuThdRwLtStFrwdBkwdPos_Val/1 -> ModeAdjustRunnable_sys/51(IfVeSMSuThdRwLtStFrwdBkwdPos_Val_read)
  IfVeSMSuThdRwLtStFrwdBkwdPosV_Val/1 -> ModeAdjustRunnable_sys/52(IfVeSMSuThdRwLtStFrwdBkwdPosV_Val_read)
  IfVeSMSuThdRwRStFrwdBkwdPos_Val/1 -> ModeAdjustRunnable_sys/53(IfVeSMSuThdRwRStFrwdBkwdPos_Val_read)
  IfVeSMSuThdRwRtStBkReclnUpwdDnwdPos_Val/1 -> ModeAdjustRunnable_sys/54(IfVeSMSuThdRwRtStBkReclnUpwdDnwdPos_Val_read)
  IfVeSMSuThdRwRtStBkReclnUpwdDnwdPosV_Val/1 -> ModeAdjustRunnable_sys/55(IfVeSMSuThdRwRtStBkReclnUpwdDnwdPosV_Val_read)
  IfVeSMSuThdRwRtStCshnFldUpwdDnwdPos_Val/1 -> ModeAdjustRunnable_sys/56(IfVeSMSuThdRwRtStCshnFldUpwdDnwdPos_Val_read)
  IfVeSMSuThdRwRtStCshnFldUpwdDnwdPosV_Val/1 -> ModeAdjustRunnable_sys/57(IfVeSMSuThdRwRtStCshnFldUpwdDnwdPosV_Val_read)
  IfVeSMSuThdRwRtStFrwdBkwdPosV_Val/1 -> ModeAdjustRunnable_sys/58(IfVeSMSuThdRwRtStFrwdBkwdPosV_Val_read)
  ModeAdjustRunnable_sys/1(IfVeSMSbDrvStRclCmdSrv_Val_write) -> IfVeSMSbDrvStRclCmdSrv_Val/1
  ModeAdjustRunnable_sys/2(IfVeSMSbSecRwRtStRclCmdSrv_Val_write) -> IfVeSMSbSecRwRtStRclCmdSrv_Val/1
  ModeAdjustRunnable_sys/3(IfVeSMSbThdRwLtStRclCmdSrv_Val_write) -> IfVeSMSbThdRwLtStRclCmdSrv_Val/1
  ModeAdjustRunnable_sys/4(IfVeSMSbThdRwRtStRclCmdSrv_Val_write) -> IfVeSMSbThdRwRtStRclCmdSrv_Val/1
  ModeAdjustRunnable_sys/5(IfVeSMSuDrvStBkReclnUpwdDnwdTrgtPos_Val_write) -> IfVeSMSuDrvStBkReclnUpwdDnwdTrgtPos_Val/1
  ModeAdjustRunnable_sys/6(IfVeSMSuDrvStCshnFrntUpwdDnwdTrgtPos_Val_write) -> IfVeSMSuDrvStCshnFrntUpwdDnwdTrgtPos_Val/1
  ModeAdjustRunnable_sys/7(IfVeSMSuDrvStCshnRrUpwdDnwdTrgtPos_Val_write) -> IfVeSMSuDrvStCshnRrUpwdDnwdTrgtPos_Val/1
  ModeAdjustRunnable_sys/8(IfVeSMSuDrvStFrwdBkwdTrgtPos_Val_write) -> IfVeSMSuDrvStFrwdBkwdTrgtPos_Val/1
  ModeAdjustRunnable_sys/9(IfVeSMSuDrvStFtUpwdDnwdTrgtPos_Val_write) -> IfVeSMSuDrvStFtUpwdDnwdTrgtPos_Val/1
  ModeAdjustRunnable_sys/10(IfVeSMSuPassStBkReclnUpwdDnwdTrgtPos_Val_write) -> IfVeSMSuPassStBkReclnUpwdDnwdTrgtPos_Val/1
  ModeAdjustRunnable_sys/11(IfVeSMSuPassStCshnFrntUpwdDnwdTrgtPos_Val_write) -> IfVeSMSuPassStCshnFrntUpwdDnwdTrgtPos_Val/1
  ModeAdjustRunnable_sys/12(IfVeSMSuPassStCshnRrUpwdDnwdTrgtPos_Val_write) -> IfVeSMSuPassStCshnRrUpwdDnwdTrgtPos_Val/1
  ModeAdjustRunnable_sys/13(IfVeSMSuPassStFrwdBkwdTrgtPos_Val_write) -> IfVeSMSuPassStFrwdBkwdTrgtPos_Val/1
  ModeAdjustRunnable_sys/14(IfVeSMSuPassStFtUpwdDnwdTrgtPos_Val_write) -> IfVeSMSuPassStFtUpwdDnwdTrgtPos_Val/1
  ModeAdjustRunnable_sys/15(IfVeSMSuPassStRclCmdSrv_Val_write) -> IfVeSMSuPassStRclCmdSrv_Val/1
  ModeAdjustRunnable_sys/16(IfVeSMSuSecRwLtStBkReclnUpwdDnwdTrgtPos_Val_write) -> IfVeSMSuSecRwLtStBkReclnUpwdDnwdTrgtPos_Val/1
  ModeAdjustRunnable_sys/17(IfVeSMSuSecRwLtStFrwdBkwdTrgtPos_Val_write) -> IfVeSMSuSecRwLtStFrwdBkwdTrgtPos_Val/1
  ModeAdjustRunnable_sys/18(IfVeSMSuSecRwLtStHdrstUpwdDnwdTrgtPos_Val_write) -> IfVeSMSuSecRwLtStHdrstUpwdDnwdTrgtPos_Val/1
  ModeAdjustRunnable_sys/19(IfVeSMSuSecRwLtStLgrstUpwdDnwdTrgtPos_Val_write) -> IfVeSMSuSecRwLtStLgrstUpwdDnwdTrgtPos_Val/1
  ModeAdjustRunnable_sys/20(IfVeSMSuSecRwLtStLtwdRtwdTrgtPos_Val_write) -> IfVeSMSuSecRwLtStLtwdRtwdTrgtPos_Val/1
  ModeAdjustRunnable_sys/21(IfVeSMSuSecRwLtStRclCmdSrv_Val_write) -> IfVeSMSuSecRwLtStRclCmdSrv_Val/1
  ModeAdjustRunnable_sys/22(IfVeSMSuSecRwRtStBkReclnUpwdDnwdTrgtPos_Val_write) -> IfVeSMSuSecRwRtStBkReclnUpwdDnwdTrgtPos_Val/1
  ModeAdjustRunnable_sys/23(IfVeSMSuSecRwRtStFrwdBkwdTrgtPos_Val_write) -> IfVeSMSuSecRwRtStFrwdBkwdTrgtPos_Val/1
  ModeAdjustRunnable_sys/24(IfVeSMSuSecRwRtStHdrstUpwdDnwdTrgtPos_Val_write) -> IfVeSMSuSecRwRtStHdrstUpwdDnwdTrgtPos_Val/1
  ModeAdjustRunnable_sys/25(IfVeSMSuSecRwRtStLgrstUpwdDnwdTrgtPos_Val_write) -> IfVeSMSuSecRwRtStLgrstUpwdDnwdTrgtPos_Val/1
  ModeAdjustRunnable_sys/26(IfVeSMSuSecRwRtStLtwdRtwdTrgtPos_Val_write) -> IfVeSMSuSecRwRtStLtwdRtwdTrgtPos_Val/1
  ModeAdjustRunnable_sys/27(IfVeSMSuThdRwLtStBkReclnUpwdDnwdTrgtPos_Val_write) -> IfVeSMSuThdRwLtStBkReclnUpwdDnwdTrgtPos_Val/1
  ModeAdjustRunnable_sys/28(IfVeSMSuThdRwLtStCshnFldUpwdDnwdTrgtPos_Val_write) -> IfVeSMSuThdRwLtStCshnFldUpwdDnwdTrgtPos_Val/1
  ModeAdjustRunnable_sys/29(IfVeSMSuThdRwLtStFrwdBkwdTrgtPos_Val_write) -> IfVeSMSuThdRwLtStFrwdBkwdTrgtPos_Val/1
  ModeAdjustRunnable_sys/30(IfVeSMSuThdRwRtStBkReclnUpwdDnwdTrgtPos_Val_write) -> IfVeSMSuThdRwRtStBkReclnUpwdDnwdTrgtPos_Val/1
  ModeAdjustRunnable_sys/31(IfVeSMSuThdRwRtStCshnFldUpwdDnwdTrgtPos_Val_write) -> IfVeSMSuThdRwRtStCshnFldUpwdDnwdTrgtPos_Val/1
  ModeAdjustRunnable_sys/32(IfVeSMSuThdRwRtStFrwdBkwdTrgtPos_Val_write) -> IfVeSMSuThdRwRtStFrwdBkwdTrgtPos_Val/1
  ModeAdjustRunnable_sys/33(isAcsMdEntryArrivedAtTargetPos_Val_write) -> isAcsMdEntryArrivedAtTargetPos_Val/1
  ModeAdjustRunnable_sys/34(isAcsMdEntryDoneFailed_Val_write) -> isAcsMdEntryDoneFailed_Val/1
  ModeAdjustRunnable_sys/35(isAcsMdEntryDoneOK_Val_write) -> isAcsMdEntryDoneOK_Val/1
  ModeAdjustRunnable_sys/36(isAcsMdExtArrivedAtTargetPos_Val_write) -> isAcsMdExtArrivedAtTargetPos_Val/1
  ModeAdjustRunnable_sys/37(isAcsMdExtDoneFailed_Val_write) -> isAcsMdExtDoneFailed_Val/1
  ModeAdjustRunnable_sys/38(isAcsMdExtDoneOK_Val_write) -> isAcsMdExtDoneOK_Val/1
  ModeAdjustRunnable_sys/39(isLfLugArrivedAtTargetPos_Val_write) -> isLfLugArrivedAtTargetPos_Val/1
  ModeAdjustRunnable_sys/40(isLfLugDoneFailed_Val_write) -> isLfLugDoneFailed_Val/1
  ModeAdjustRunnable_sys/41(isLfLugDoneOK_Val_write) -> isLfLugDoneOK_Val/1
  ModeAdjustRunnable_sys/42(isLfRecoveryArrivedAtTargetPos_Val_write) -> isLfRecoveryArrivedAtTargetPos_Val/1
  ModeAdjustRunnable_sys/43(isLfRecoveryDoneFailed_Val_write) -> isLfRecoveryDoneFailed_Val/1
  ModeAdjustRunnable_sys/44(isLfRecoveryDoneOK_Val_write) -> isLfRecoveryDoneOK_Val/1
  ModeAdjustRunnable_sys/45(isLfVipArrivedAtTargetPos_Val_write) -> isLfVipArrivedAtTargetPos_Val/1
  ModeAdjustRunnable_sys/46(isLfVipDoneFailed_Val_write) -> isLfVipDoneFailed_Val/1
  ModeAdjustRunnable_sys/47(isLfVipDoneOK_Val_write) -> isLfVipDoneOK_Val/1
  ModeAdjustRunnable_sys/48(isRtLugArrivedAtTargetPos_Val_write) -> isRtLugArrivedAtTargetPos_Val/1
  ModeAdjustRunnable_sys/49(isRtLugDoneFailed_Val_write) -> isRtLugDoneFailed_Val/1
  ModeAdjustRunnable_sys/50(isRtLugDoneOK_Val_write) -> isRtLugDoneOK_Val/1
  ModeAdjustRunnable_sys/51(isRtRecoveryArrivedAtTargetPos_Val_write) -> isRtRecoveryArrivedAtTargetPos_Val/1
  ModeAdjustRunnable_sys/52(isRtRecoveryDoneFailed_Val_write) -> isRtRecoveryDoneFailed_Val/1
  ModeAdjustRunnable_sys/53(isRtRecoveryDoneOK_Val_write) -> isRtRecoveryDoneOK_Val/1
  ModeAdjustRunnable_sys/54(isRtVipArrivedAtTargetPos_Val_write) -> isRtVipArrivedAtTargetPos_Val/1
  ModeAdjustRunnable_sys/55(isRtVipDoneFailed_Val_write) -> isRtVipDoneFailed_Val/1
  ModeAdjustRunnable_sys/56(isRtVipDoneOK_Val_write) -> isRtVipDoneOK_Val/1
  ModeAdjustRunnable/1 -> ModeAdjustRunnable_sys/Trigger
  IfVeSMSeNotThdRowRtSeaOccStat_Val/1 -> ModeAdjustRunnable_sys/59(IfVeSMSeNotThdRowRtSeaOccStat_Val_read)
  IfVeSMSeNotThdRwCtStOccStat_Val/1 -> ModeAdjustRunnable_sys/60(IfVeSMSeNotThdRwCtStOccStat_Val_read)
  IfVeSMSeNotThdRwLtStOccStat_Val/1 -> ModeAdjustRunnable_sys/61(IfVeSMSeNotThdRwLtStOccStat_Val_read)
  ModeAdjustRunnable_sys/57(IfVeSMSuSecRwLtStArmScrnTrgtPos_Val_write) -> IfVeSMSuSecRwLtStArmScrnTrgtPos_Val/1
  ModeAdjustRunnable_sys/58(IfVeSMSuSecRwRtStArmScrnTrgtPos_Val_write) -> IfVeSMSuSecRwRtStArmScrnTrgtPos_Val/1
  modestate32_Val/1 -> ModeAdjustRunnable_sys/62(modestate32_Val_read)
  PwrMdChked_Val/1 -> ModeAdjustRunnable_sys/63(PwrMdChked_Val_read)
  IfVeSMSbDrvStBkReclnUpwdDnwdMovConfig_Val/1 -> ModeAdjustRunnable_sys/64(IfVeSMSbDrvStBkReclnUpwdDnwdMovConfig_Val_read)
  IfVeSMSbDrvStFrwdBkwdMovConfig_Val/1 -> ModeAdjustRunnable_sys/65(IfVeSMSbDrvStFrwdBkwdMovConfig_Val_read)
  IfVeSMSbDrvStFtUpwdDnwdMovConfig_Val/1 -> ModeAdjustRunnable_sys/66(IfVeSMSbDrvStFtUpwdDnwdMovConfig_Val_read)
  IfVeSMSbPassStBkReclnUpwdDnwdMovConfig_Val/1 -> ModeAdjustRunnable_sys/67(IfVeSMSbPassStBkReclnUpwdDnwdMovConfig_Val_read)
  IfVeSMSbPassStFrwdBkwdMovConfig_Val/1 -> ModeAdjustRunnable_sys/68(IfVeSMSbPassStFrwdBkwdMovConfig_Val_read)
  IfVeSMSbPassStFtUpwdDnwdMovConfig_Val/1 -> ModeAdjustRunnable_sys/69(IfVeSMSbPassStFtUpwdDnwdMovConfig_Val_read)
  IfVeSMSbSecRwRtStBkReclnUpwdDnwdMovConfig_Val/1 -> ModeAdjustRunnable_sys/70(IfVeSMSbSecRwRtStBkReclnUpwdDnwdMovConfig_Val_read)
  IfVeSMSbSecRwRtStBlstOtwdInwdMovConfig_Val/1 -> ModeAdjustRunnable_sys/71(IfVeSMSbSecRwRtStBlstOtwdInwdMovConfig_Val_read)
  IfVeSMSbSecRwRtStFrwdBkwdMovConfig_Val/1 -> ModeAdjustRunnable_sys/72(IfVeSMSbSecRwRtStFrwdBkwdMovConfig_Val_read)
  IfVeSMSbSecRwRtStLgrstUpwdMovConfig_Val/1 -> ModeAdjustRunnable_sys/73(IfVeSMSbSecRwRtStLgrstUpwdMovConfig_Val_read)
  IfVeSMSbSecRwRtStLtwdRtwdMovConfig_Val/1 -> ModeAdjustRunnable_sys/74(IfVeSMSbSecRwRtStLtwdRtwdMovConfig_Val_read)
  IfVeSMSbThdRwLtStBkReclnUpwdDnwdMovConfig_Val/1 -> ModeAdjustRunnable_sys/75(IfVeSMSbThdRwLtStBkReclnUpwdDnwdMovConfig_Val_read)
  IfVeSMSbThdRwLtStCshnFldUpwdDnwdMovConfig_Val/1 -> ModeAdjustRunnable_sys/76(IfVeSMSbThdRwLtStCshnFldUpwdDnwdMovConfig_Val_read)
  IfVeSMSbThdRwLtStFrwdBkwdMovConfig_Val/1 -> ModeAdjustRunnable_sys/77(IfVeSMSbThdRwLtStFrwdBkwdMovConfig_Val_read)
  IfVeSMSbThdRwRtStBkReclnUpwdDnwdMovConfig_Val/1 -> ModeAdjustRunnable_sys/78(IfVeSMSbThdRwRtStBkReclnUpwdDnwdMovConfig_Val_read)
  IfVeSMSbThdRwRtStCshnFldUpwdDnwdMovConfig_Val/1 -> ModeAdjustRunnable_sys/79(IfVeSMSbThdRwRtStCshnFldUpwdDnwdMovConfig_Val_read)
  IfVeSMSbThdRwRtStFrwdBkwdMovConfig_Val/1 -> ModeAdjustRunnable_sys/80(IfVeSMSbThdRwRtStFrwdBkwdMovConfig_Val_read)
  IfVeSMSuRrLtStFtUpwdDnwdPos_Val/1 -> ModeAdjustRunnable_sys/81(IfVeSMSuRrLtStFtUpwdDnwdPos_Val_read)
  IfVeSMSuRrLtStFtUpwdDnwdPosV_Val/1 -> ModeAdjustRunnable_sys/82(IfVeSMSuRrLtStFtUpwdDnwdPosV_Val_read)
  IfVeSMSuRrRtStFtUpwdDnwdPos_Val/1 -> ModeAdjustRunnable_sys/83(IfVeSMSuRrRtStFtUpwdDnwdPos_Val_read)
  IfVeSMSuRrRtStFtUpwdDnwdPosV_Val/1 -> ModeAdjustRunnable_sys/84(IfVeSMSuRrRtStFtUpwdDnwdPosV_Val_read)
  IfVeSMSuSecRwLtStLgrstOtwdInwdPos_Val/1 -> ModeAdjustRunnable_sys/85(IfVeSMSuSecRwLtStLgrstOtwdInwdPos_Val_read)
  IfVeSMSuSecRwLtStLgrstOtwdInwdPosV_Val/1 -> ModeAdjustRunnable_sys/86(IfVeSMSuSecRwLtStLgrstOtwdInwdPosV_Val_read)
  IfVeSMSuSecRwRtStLgrstOtwdInwdPos_Val/1 -> ModeAdjustRunnable_sys/87(IfVeSMSuSecRwRtStLgrstOtwdInwdPos_Val_read)
  IfVeSMSuSecRwRtStLgrstOtwdInwdPosV_Val/1 -> ModeAdjustRunnable_sys/88(IfVeSMSuSecRwRtStLgrstOtwdInwdPosV_Val_read)
  ModeAdjustRunnable_sys/59(IfVeSMSuRrLtStFtUpwdDnwdTrgtPos_Val_write) -> IfVeSMSuRrLtStFtUpwdDnwdTrgtPos_Val/1
  ModeAdjustRunnable_sys/60(IfVeSMSuRrRtStFtUpwdDnwdTrgtPos_Val_write) -> IfVeSMSuRrRtStFtUpwdDnwdTrgtPos_Val/1
  ModeAdjustRunnable_sys/61(IfVeSMSuSecRwLtStLgrstOtwdInwdTrgtPos_Val_write) -> IfVeSMSuSecRwLtStLgrstOtwdInwdTrgtPos_Val/1
  ModeAdjustRunnable_sys/62(IfVeSMSuSecRwRtStLgrstOtwdInwdTrgtPos_Val_write) -> IfVeSMSuSecRwRtStLgrstOtwdInwdTrgtPos_Val/1
  ModeAdjustRunnable_sys/63(isINTMArrivedAtTargetPos_Val_write) -> isINTMArrivedAtTargetPos_Val/1
  ModeAdjustRunnable_sys/64(isINTMDoneFailed_Val_write) -> isINTMDoneFailed_Val/1
  ModeAdjustRunnable_sys/65(isINTMDoneOK_Val_write) -> isINTMDoneOK_Val/1
  ModeAdjustRunnable_sys/66(isLfFamlyArrivedAtTargetPos_Val_write) -> isLfFamlyArrivedAtTargetPos_Val/1
  ModeAdjustRunnable_sys/67(isLfFamlyDoneFailed_Val_write) -> isLfFamlyDoneFailed_Val/1
  ModeAdjustRunnable_sys/68(isLfFamlyDoneOK_Val_write) -> isLfFamlyDoneOK_Val/1
  ModeAdjustRunnable_sys/69(isLfLyArrivedAtTargetPos_Val_write) -> isLfLyArrivedAtTargetPos_Val/1
  ModeAdjustRunnable_sys/70(isLfLyDoneFailed_Val_write) -> isLfLyDoneFailed_Val/1
  ModeAdjustRunnable_sys/71(isLfLyDoneOK_Val_write) -> isLfLyDoneOK_Val/1
  ModeAdjustRunnable_sys/72(isRfFamlyDoneFailed_Val_write) -> isRfFamlyDoneFailed_Val/1
  ModeAdjustRunnable_sys/73(isRfFamlyDoneOK_Val_write) -> isRfFamlyDoneOK_Val/1
  ModeAdjustRunnable_sys/74(isRtFamlyArrivedAtTargetPos_Val_write) -> isRtFamlyArrivedAtTargetPos_Val/1
  ModeAdjustRunnable_sys/75(isRtLyArrivedAtTargetPos_Val_write) -> isRtLyArrivedAtTargetPos_Val/1
  ModeAdjustRunnable_sys/76(isRtLyDoneFailed_Val_write) -> isRtLyDoneFailed_Val/1
  ModeAdjustRunnable_sys/77(isRtLyDoneOK_Val_write) -> isRtLyDoneOK_Val/1
  IfVeSMSbSecRwRtSLgrstExpdMovConfig_Val/1 -> ModeAdjustRunnable_sys/89(IfVeSMSbSecRwRtSLgrstExpdMovConfig_Val_read)
  IfVeSMSbSecRwRtStFtrstMovConfig_Val/1 -> ModeAdjustRunnable_sys/90(IfVeSMSbSecRwRtStFtrstMovConfig_Val_read)
  IfVeSMSbSecRwRtStHdUpwdDnwdMovConfig_Val/1 -> ModeAdjustRunnable_sys/91(IfVeSMSbSecRwRtStHdUpwdDnwdMovConfig_Val_read)
  IfVeSMSbThdRwLtStFrwdCmdSrv_Val/1 -> ModeAdjustRunnable_sys/92(IfVeSMSbThdRwLtStFrwdCmdSrv_Val_read)
  IfVeSMSbThdRwRtStFrwdCmdSrv_Val/1 -> ModeAdjustRunnable_sys/93(IfVeSMSbThdRwRtStFrwdCmdSrv_Val_read)
  IfVeSMSbSecRwRtStHdrstFrwdBkwdMovConfig_Val/1 -> ModeAdjustRunnable_sys/94(IfVeSMSbSecRwRtStHdrstFrwdBkwdMovConfig_Val_read)
  IfVeSMSuSecRwLtStHdrstFrwdBkwdPos_Val/1 -> ModeAdjustRunnable_sys/95(IfVeSMSuSecRwLtStHdrstFrwdBkwdPos_Val_read)
  IfVeSMSuSecRwLtStHdrstFrwdBkwdPosV_Val/1 -> ModeAdjustRunnable_sys/96(IfVeSMSuSecRwLtStHdrstFrwdBkwdPosV_Val_read)
  IfVeSMSuSecRwRtStHdrstFrwdBkwdPos_Val/1 -> ModeAdjustRunnable_sys/97(IfVeSMSuSecRwRtStHdrstFrwdBkwdPos_Val_read)
  IfVeSMSuSecRwRtStHdrstFrwdBkwdPosV_Val/1 -> ModeAdjustRunnable_sys/98(IfVeSMSuSecRwRtStHdrstFrwdBkwdPosV_Val_read)
  ModeAdjustRunnable_sys/78(IfVeSMSuSecRwLtStHdrstFrwdBkwdTrgtPos_Val_write) -> IfVeSMSuSecRwLtStHdrstFrwdBkwdTrgtPos_Val/1
  ModeAdjustRunnable_sys/79(IfVeSMSuSecRwRtStHdrstFrwdBkwdTrgtPos_Val_write) -> IfVeSMSuSecRwRtStHdrstFrwdBkwdTrgtPos_Val/1
  IfVeSMSeNotSecRowLeSeaOccStat_Val/1 -> ModeAdjustRunnable_sys/99(IfVeSMSeNotSecRowLeSeaOccStat_Val_read)
  IfVeSMSeNotSecRowRtSeaOccStat_Val/1 -> ModeAdjustRunnable_sys/100(IfVeSMSeNotSecRowRtSeaOccStat_Val_read)
  ModeAdjustRunnable_sys/80(IfVeSMSeSecRwLtStMdRclLgSldSpdCrl_Val_write) -> IfVeSMSeSecRwLtStMdRclLgSldSpdCrl_Val/1
  ModeAdjustRunnable_sys/81(IfVeSMSeSecRwRtStMdRclLgSldSpdCrl_Val_write) -> IfVeSMSeSecRwRtStMdRclLgSldSpdCrl_Val/1
  ModeAdjustRunnable_sys/82(IfVeSMSeThdRwLtStMdRclLgSldSpdCrl_Val_write) -> IfVeSMSeThdRwLtStMdRclLgSldSpdCrl_Val/1
  ModeAdjustRunnable_sys/83(IfVeSMSeThdRwRtStMdRclLgSldSpdCrl_Val_write) -> IfVeSMSeThdRwRtStMdRclLgSldSpdCrl_Val/1
  ModeAdjustRunnable_sys/84(isINTMRArrivedAtTargetPos_Val_write) -> isINTMRArrivedAtTargetPos_Val/1
  ModeAdjustRunnable_sys/85(isINTMRDoneFailed_Val_write) -> isINTMRDoneFailed_Val/1
  ModeAdjustRunnable_sys/86(isINTMRDoneOK_Val_write) -> isINTMRDoneOK_Val/1
  ModeAdjustRunnable_sys/87(isLgrstCloseLArrivedAtTargetPos_Val_write) -> isLgrstCloseLArrivedAtTargetPos_Val/1
  ModeAdjustRunnable_sys/88(isLgrstCloseLDoneFailed_Val_write) -> isLgrstCloseLDoneFailed_Val/1
  ModeAdjustRunnable_sys/89(isLgrstCloseLDoneOK_Val_write) -> isLgrstCloseLDoneOK_Val/1
  ModeAdjustRunnable_sys/90(isLgrstCloseRArrivedAtTargetPos_Val_write) -> isLgrstCloseRArrivedAtTargetPos_Val/1
  ModeAdjustRunnable_sys/91(isLgrstCloseRDoneFailed_Val_write) -> isLgrstCloseRDoneFailed_Val/1
  ModeAdjustRunnable_sys/92(isLgrstCloseRDoneOK_Val_write) -> isLgrstCloseRDoneOK_Val/1
  ModeAdjustRunnable_sys/93(isLgrstOpenLArrivedAtTargetPos_Val_write) -> isLgrstOpenLArrivedAtTargetPos_Val/1
  ModeAdjustRunnable_sys/94(isLgrstOpenLDoneFailed_Val_write) -> isLgrstOpenLDoneFailed_Val/1
  ModeAdjustRunnable_sys/95(isLgrstOpenLDoneOK_Val_write) -> isLgrstOpenLDoneOK_Val/1
  ModeAdjustRunnable_sys/96(isLgrstOpenRArrivedAtTargetPos_Val_write) -> isLgrstOpenRArrivedAtTargetPos_Val/1
  ModeAdjustRunnable_sys/97(isLgrstOpenRDoneFailed_Val_write) -> isLgrstOpenRDoneFailed_Val/1
  ModeAdjustRunnable_sys/98(isLgrstOpenRDoneOK_Val_write) -> isLgrstOpenRDoneOK_Val/1
  IfVeSMSeStNumConfig_Val/1 -> ModeAdjustRunnable_sys/101(IfVeSMSeStNumConfig_Val_read)
